simulink library "equationsOfMotionLib"  (R2021b)
settings: Solver=VariableStepAuto  StartTime=0.0  StopTime=10.0  RelTol=1e-3
settings Model: Creator=mat  LastModifiedBy=mat

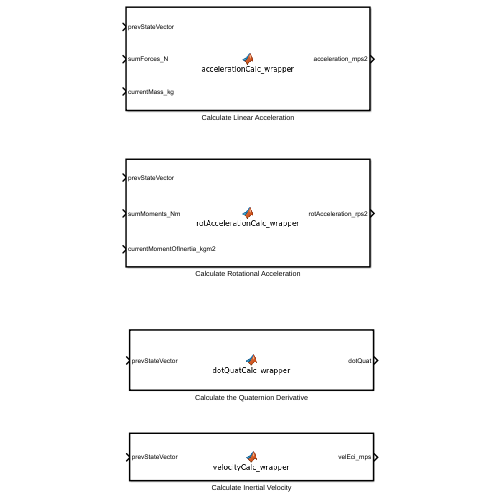
[thumbnail: Simulink's stored preview of the top-level diagram]
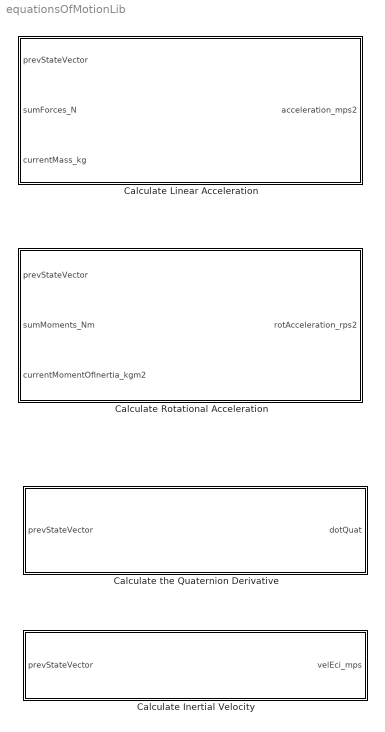
== system equationsOfMotionLib ==
  Calculate Inertial Velocity : MATLAB Function  TreatAsAtomicUnit=on
  Calculate Linear Acceleration : MATLAB Function  TreatAsAtomicUnit=on
  Calculate Rotational Acceleration : MATLAB Function  TreatAsAtomicUnit=on
  Calculate the Quaternion Derivative : MATLAB Function  TreatAsAtomicUnit=on

== matlab function equationsOfMotionLib/Calculate Linear Acceleration ==
  data: prevStateVector input Bus: StateVector; acceleration_mps2 output; sumForces_N input; currentMass_kg input
function acceleration_mps2 = accelerationCalc_wrapper(prevStateVector, sumForces_N, currentMass_kg)
% This function is just a wrapper. To easily open the real function, right
% click velocityDotCalc below, and click open. 

    acceleration_mps2 = accelerationCalc(prevStateVector, sumForces_N, currentMass_kg);

end

== matlab function equationsOfMotionLib/Calculate the Quaternion Derivative ==
  data: prevStateVector input Bus: StateVector; dotQuat output
function dotQuat = dotQuatCalc_wrapper(prevStateVector)

dotQuat = dotQuatCalc(prevStateVector);

end

== matlab function equationsOfMotionLib/Calculate Inertial Velocity ==
  data: prevStateVector input Bus: StateVector; velEci_mps output
function velEci_mps  = velocityCalc_wrapper(prevStateVector)

[velEci_mps] = velocityCalc(prevStateVector);

end

== matlab function equationsOfMotionLib/Calculate Rotational Acceleration ==
  data: prevStateVector input Bus: StateVector; rotAcceleration_rps2 output; sumMoments_Nm input; currentMomentOfInertia_kgm2 input
function rotAcceleration_rps2 = rotAccelerationCalc_wrapper(prevStateVector, sumMoments_Nm, currentMomentOfInertia_kgm2)

rotAcceleration_rps2 = rotAccelerationCalc(prevStateVector, sumMoments_Nm, currentMomentOfInertia_kgm2);

end
